simulink subsystem "MOV_05_SS"  (R2022a)
settings: Solver=VariableStepAuto  StartTime=0.0  StopTime=10.0  RelTol=1e-3
libraries: hdlBasic x31
settings Model: Creator=sebas  LastModifiedBy=viktor

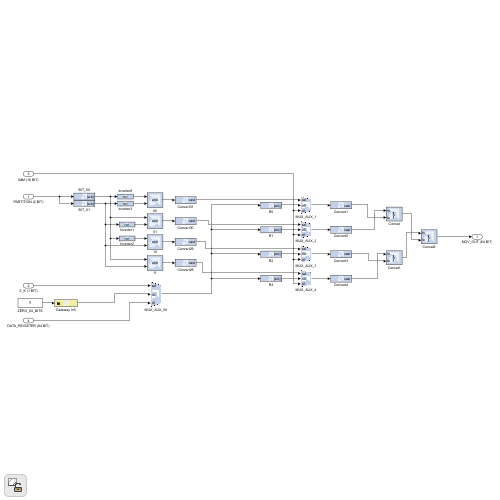
[thumbnail: Simulink's stored preview of the top-level diagram]
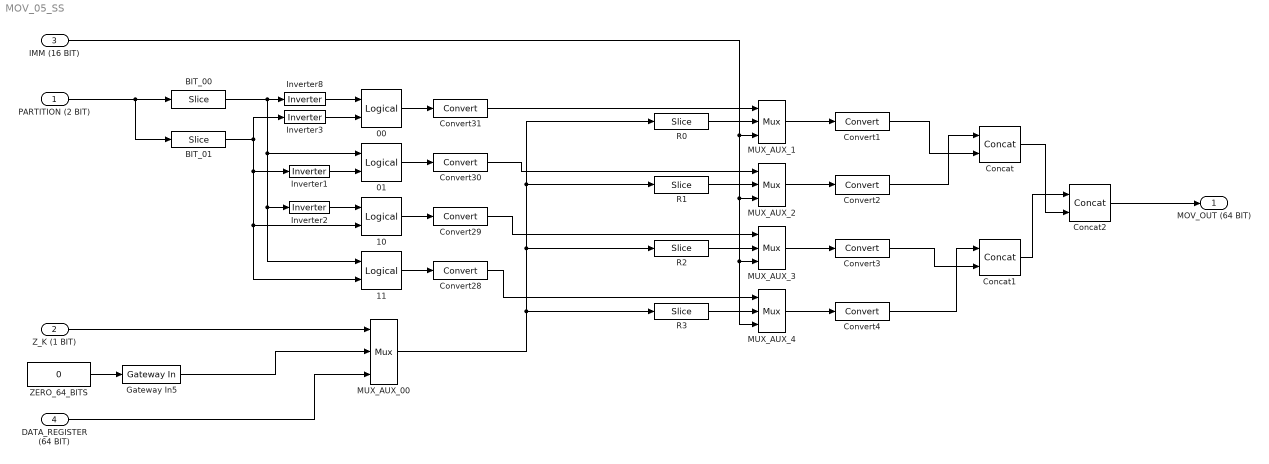
== system MOV_05_SS ==
  PARTITION (2 BIT) : Inport
  Z_K (1 BIT) : Inport  Port=2
  IMM (16 BIT) : Inport  Port=3
  DATA_REGISTER (64 BIT) : Inport  Port=4
  00 : hdlBasic/Logical  logical_function=AND  inputs=2  en=off  latency=0  precision=Full  arith_type=Unsigned  n_bits=16  bin_pt=0  align_bp=on  overflow=[]  quantization=[]  XmcBlockStatus=1  maskContainerNames=tabcontainer1  block_type=logical  block_config=sysgen:Logical_config
  01 : hdlBasic/Logical  logical_function=AND  inputs=2  en=off  latency=0  precision=Full  arith_type=Unsigned  n_bits=16  bin_pt=0  align_bp=on  overflow=[]  quantization=[]  XmcBlockStatus=1  maskContainerNames=tabcontainer1  block_type=logical  block_config=sysgen:Logical_config
  10 : hdlBasic/Logical  logical_function=AND  inputs=2  en=off  latency=0  precision=Full  arith_type=Unsigned  n_bits=16  bin_pt=0  align_bp=on  overflow=[]  quantization=[]  XmcBlockStatus=1  maskContainerNames=tabcontainer1  block_type=logical  block_config=sysgen:Logical_config
  11 : hdlBasic/Logical  logical_function=AND  inputs=2  en=off  latency=0  precision=Full  arith_type=Unsigned  n_bits=16  bin_pt=0  align_bp=on  overflow=[]  quantization=[]  XmcBlockStatus=1  maskContainerNames=tabcontainer1  block_type=logical  block_config=sysgen:Logical_config
  BIT_00 : hdlBasic/Slice  nbits=1  boolean_output=off  mode=Lower Bit Location + Width  bit1=-3  base1=MSB of Input  bit0=0  base0=LSB of Input  XmcBlockStatus=1  maskContainerNames=group1  block_type=slice  block_config=sysgen:Slice_config
  BIT_01 : hdlBasic/Slice  nbits=1  boolean_output=off  mode=Lower Bit Location + Width  bit1=-2  base1=MSB of Input  bit0=1  base0=LSB of Input  XmcBlockStatus=1  maskContainerNames=group1  block_type=slice  block_config=sysgen:Slice_config
  Concat : hdlBasic/Concat  num_inputs=2  XmcBlockStatus=1  maskContainerNames=group1  block_type=concat  block_config=sysgen:Concat_config
  Concat1 : hdlBasic/Concat  num_inputs=2  XmcBlockStatus=1  maskContainerNames=group1  block_type=concat  block_config=sysgen:Concat_config
  Concat2 : hdlBasic/Concat  num_inputs=2  XmcBlockStatus=1  maskContainerNames=group1  block_type=concat  block_config=sysgen:Concat_config
  Convert{1..4} (4 alike) : hdlBasic/Convert  gui_display_data_type=Fixed-point  arith_type=Unsigned  n_bits=16  bin_pt=0  float_type=Single  exp_bits=8  fraction_bits=24  quantization=Truncate  overflow=Wrap  en=off  latency=0  pipeline=off  XmcBlockStatus=1  maskContainerNames=group2  block_type=convert  block_config=sysgen:Convert_config  block_width=595  block_height=885
  Convert{28..31} (4 alike) : hdlBasic/Convert  gui_display_data_type=Fixed-point  arith_type=Unsigned  n_bits=1  bin_pt=0  float_type=Single  exp_bits=8  fraction_bits=24  quantization=Truncate  overflow=Wrap  en=off  latency=0  pipeline=off  XmcBlockStatus=1  maskContainerNames=group2  block_type=convert  block_config=sysgen:Convert_config  block_width=595  block_height=885
  Gateway In5 : hdlBasic/Gateway In  gui_display_data_type=Fixed-point  arith_type=Unsigned  n_bits=64  bin_pt=0  preci_type=Single  exp_width=8  frac_width=24  rows=1  columns=1  quantization="Round  (unbiased: +/- Inf)"  overflow=Saturate  period=1  UseAsADC=off  ADCChannel='1'  interface=None  automatic_assignment=on  address_offset=hex2dec('00')  intf_name=''  intf_description=''  default_value=0  timing_constraint=None  locs_specified=off  LOCs={}  io_standard={}  inherit_from_input=off  hdl_port=on  XmcBlockStatus=1  maskContainerNames=group4  block_type=gatewayin  block_config=sysgen:gateway_in_config  block_width_w=590  block_height_w=620  block_width=640  block_height=850
  Inverter{1..3,8} (4 alike) : hdlBasic/Inverter  en=off  latency=0  XmcBlockStatus=1  maskContainerNames=group2  block_type=inv  block_config=sysgen:Inverter_config
  MUX_AUX_00 : hdlBasic/Mux  inputs=2  en=off  latency=0  precision=Full  arith_type=Unsigned  n_bits=16  bin_pt=14  quantization=Truncate  overflow=Wrap  XmcBlockStatus=1  maskContainerNames=tabcontainer1  block_type=mux  block_config=sysgen:Mux_config
  MUX_AUX_{1..4} (4 alike) : hdlBasic/Mux  inputs=2  en=off  latency=0  precision=Full  arith_type=Unsigned  n_bits=16  bin_pt=14  quantization=Truncate  overflow=Wrap  XmcBlockStatus=1  maskContainerNames=tabcontainer1  block_type=mux  block_config=sysgen:Mux_config
  R0 : hdlBasic/Slice  nbits=16  boolean_output=off  mode=Lower Bit Location + Width  bit1=15  base1=LSB of Input  bit0=0  base0=LSB of Input  XmcBlockStatus=1  maskContainerNames=group1  block_type=slice  block_config=sysgen:Slice_config
  R1 : hdlBasic/Slice  nbits=16  boolean_output=off  mode=Lower Bit Location + Width  bit1=31  base1=LSB of Input  bit0=16  base0=LSB of Input  XmcBlockStatus=1  maskContainerNames=group1  block_type=slice  block_config=sysgen:Slice_config
  R2 : hdlBasic/Slice  nbits=16  boolean_output=off  mode=Lower Bit Location + Width  bit1=47  base1=LSB of Input  bit0=32  base0=LSB of Input  XmcBlockStatus=1  maskContainerNames=group1  block_type=slice  block_config=sysgen:Slice_config
  R3 : hdlBasic/Slice  nbits=16  boolean_output=off  mode=Lower Bit Location + Width  bit1=63  base1=LSB of Input  bit0=48  base0=LSB of Input  XmcBlockStatus=1  maskContainerNames=group1  block_type=slice  block_config=sysgen:Slice_config
  ZERO_64_BITS : Constant  Value=0
  MOV_OUT (64 BIT) : Outport
  wires:
  ZERO_64_BITS/1 -> Gateway In5/1
  00/1 -> Convert31/1
  01/1 -> Convert30/1
  Inverter8/1 -> 00/1
  Inverter3/1 -> 00/2
  BIT_01/1 -> Inverter1/1, 10/2, 11/2, Inverter3/1
  Gateway In5/1 -> MUX_AUX_00/2
  IMM (16 BIT)/1 -> MUX_AUX_1/3, MUX_AUX_2/3, MUX_AUX_3/3, MUX_AUX_4/3
  Inverter2/1 -> 10/1
  10/1 -> Convert29/1
  Inverter1/1 -> 01/2
  Convert31/1 -> MUX_AUX_1/1
  Convert28/1 -> MUX_AUX_4/1
  Convert30/1 -> MUX_AUX_2/1
  Convert29/1 -> MUX_AUX_3/1
  BIT_00/1 -> Inverter8/1, 01/1, Inverter2/1, 11/1
  DATA_REGISTER (64 BIT)/1 -> MUX_AUX_00/3
  Z_K (1 BIT)/1 -> MUX_AUX_00/1
  11/1 -> Convert28/1
  PARTITION (2 BIT)/1 -> BIT_00/1, BIT_01/1
  R1/1 -> MUX_AUX_2/2
  R2/1 -> MUX_AUX_3/2
  R3/1 -> MUX_AUX_4/2
  MUX_AUX_00/1 -> R3/1, R2/1, R1/1, R0/1
  R0/1 -> MUX_AUX_1/2
  MUX_AUX_1/1 -> Convert1/1
  MUX_AUX_2/1 -> Convert2/1
  MUX_AUX_3/1 -> Convert3/1
  MUX_AUX_4/1 -> Convert4/1
  Convert1/1 -> Concat/2
  Convert2/1 -> Concat/1
  Convert3/1 -> Concat1/2
  Convert4/1 -> Concat1/1
  Concat/1 -> Concat2/2
  Concat1/1 -> Concat2/1
  Concat2/1 -> MOV_OUT (64 BIT)/1
